simulink model "untitled"  (R2020b)
settings: Solver=FixedStepAuto  StartTime=0.0  StopTime=10.0  RelTol=1e-3
undefined symbols (not defined in the file): DiscIntNeverNeededParam
libraries: simulink x2
settings Model: Creator=xoxox  LastModifiedBy=xoxox
settings OptimizationCC: DefaultParameterBehavior=Inlined  EnhancedBackFolding=on  PassReuseOutputArgsAs=Individual arguments  ZeroExternalMemoryAtStartup=off  ZeroInternalMemoryAtStartup=off  OptimizeBlockOrder=speed  DifferentSizesBufferReuse=on  OptimizationCustomize=off  EfficientTunableParamExpr=on
settings DebuggingCC: ParameterTunabilityLossMsg=error
settings SFSimCC: MATLABDynamicMemAlloc=off
settings RTWCC: Description=Embedded Coder  SystemTargetFile=ert.tlc  GenCodeOnly=on  TemplateMakefile=ert_default_tmf  TargetLang=C++
settings CodeAppCC: ForceParamTrailComments=on  IgnoreCustomStorageClasses=off  OperatorAnnotations=on  SimulinkDataObjDesc=on  SFDataObjDesc=on  InsertBlockDesc=on
settings ERTTargetCC: TargetLangStandard=C++03 (ISO)  GenerateSampleERTMain=on  CodeInterfacePackaging=C++ class  InlinedParameterPlacement=NonHierarchical  RootIOFormat=Structure reference  ERTCustomFileTemplate=example_file_process.tlc

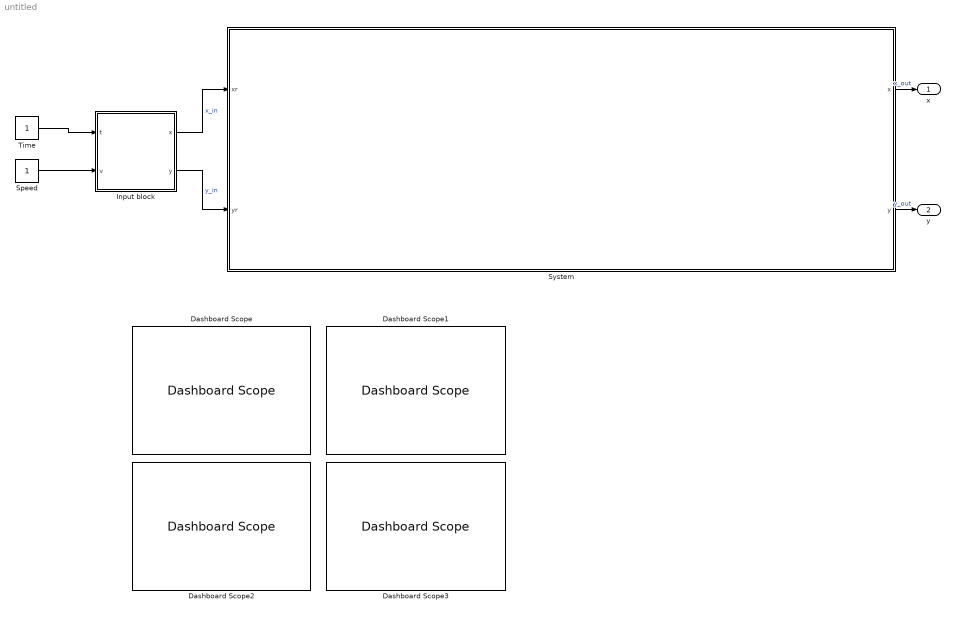
== system untitled ==
  Dashboard Scope{,1..3} (4 alike) : DashboardScope
  Input block : MATLAB Function  TreatAsAtomicUnit=on
  Speed : Constant
  System : Subsystem
  Time : Constant
  x : Outport  VectorParamsAs1DForOutWhenUnconnected=off
  y : Outport  Port=2  VectorParamsAs1DForOutWhenUnconnected=off
  wires:
  Input block/1(x) -> System/1(xr)  "x_in"
  Input block/2(y) -> System/2(yr)  "y_in"
  System/1(x) -> x/1  "x_out"
  System/2(y) -> y/1  "y_out"
  Speed/1 -> Input block/2(v)
  Time/1 -> Input block/1(t)

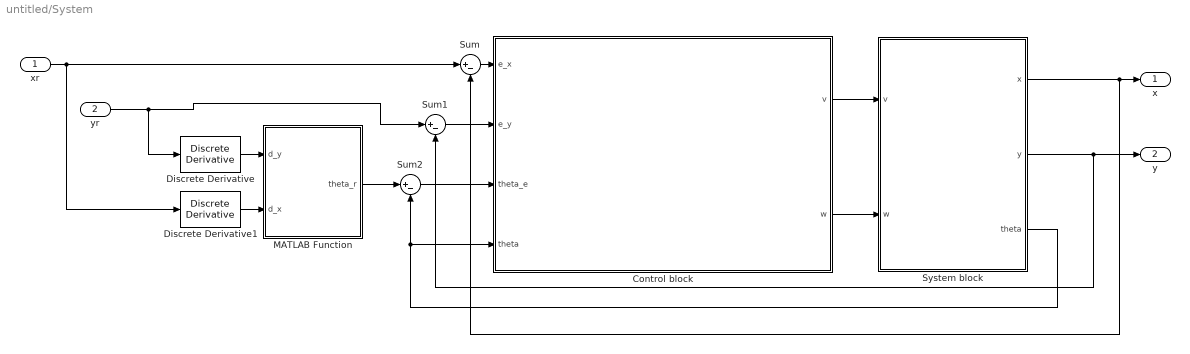
== system untitled/System ==
  xr : Inport
  yr : Inport  Port=2
  Control block : Subsystem
  Discrete Derivative : simulink/Discrete/Discrete Derivative  gainval=1.0  ICPrevScaledInput=0.0  OutMin=[]  OutMax=[]  OutDataType=fixdt(1, 16)  OutScaling=2^-10  DoSatur=off
  Discrete Derivative1 : simulink/Discrete/Discrete Derivative  gainval=1.0  ICPrevScaledInput=0.0  OutMin=[]  OutMax=[]  OutDataType=fixdt(1, 16)  OutScaling=2^-10  DoSatur=off
  MATLAB Function : MATLAB Function  TreatAsAtomicUnit=on
  Sum : Sum  Inputs=|+-
  Sum1 : Sum  Inputs=|+-
  Sum2 : Sum  Inputs=|+-
  System block : Subsystem
  x : Outport  VectorParamsAs1DForOutWhenUnconnected=off
  y : Outport  Port=2  VectorParamsAs1DForOutWhenUnconnected=off
  wires:
  Sum1/1 -> Control block/2(e_y)
  Control block/2(w) -> System block/2(w)
  Discrete Derivative/1 -> MATLAB Function/1(d_y)
  MATLAB Function/1(theta_r) -> Sum2/1
  System block/2(y) -> y/1, Sum1/2
  System block/3(theta) -> Control block/4(theta), Sum2/2
  System block/1(x) -> x/1, Sum/2
  Discrete Derivative1/1 -> MATLAB Function/2(d_x)
  Sum/1 -> Control block/1(e_x)
  Control block/1(v) -> System block/1(v)
  Sum2/1 -> Control block/3(theta_e)
  xr/1 -> Discrete Derivative1/1, Sum/1
  yr/1 -> Discrete Derivative/1, Sum1/1

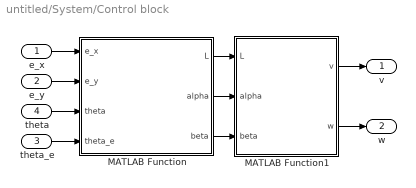
== system untitled/System/Control block ==
  e_x : Inport
  e_y : Inport  Port=2
  theta_e : Inport  Port=3
  theta : Inport  Port=4
  MATLAB Function : MATLAB Function  TreatAsAtomicUnit=on
  MATLAB Function1 : MATLAB Function  TreatAsAtomicUnit=on
  v : Outport  VectorParamsAs1DForOutWhenUnconnected=off
  w : Outport  Port=2  VectorParamsAs1DForOutWhenUnconnected=off
  wires:
  MATLAB Function1/1(v) -> v/1
  MATLAB Function1/2(w) -> w/1
  e_x/1 -> MATLAB Function/1(e_x)
  e_y/1 -> MATLAB Function/2(e_y)
  theta_e/1 -> MATLAB Function/4(theta_e)
  MATLAB Function/1(L) -> MATLAB Function1/1(L)
  MATLAB Function/2(alpha) -> MATLAB Function1/2(alpha)
  MATLAB Function/3(beta) -> MATLAB Function1/3(beta)
  theta/1 -> MATLAB Function/3(theta)

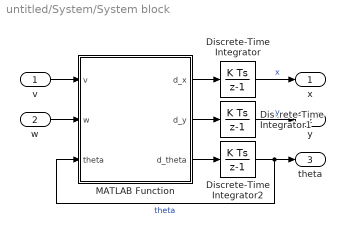
== system untitled/System/System block ==
  v : Inport
  w : Inport  Port=2
  Discrete-Time Integrator : DiscreteIntegrator  SampleTime=-1  ICPrevOutput=DiscIntNeverNeededParam  ICPrevScaledInput=DiscIntNeverNeededParam
  Discrete-Time Integrator1 : DiscreteIntegrator  SampleTime=-1  ICPrevOutput=DiscIntNeverNeededParam  ICPrevScaledInput=DiscIntNeverNeededParam
  Discrete-Time Integrator2 : DiscreteIntegrator  SampleTime=-1  ICPrevOutput=DiscIntNeverNeededParam  ICPrevScaledInput=DiscIntNeverNeededParam
  MATLAB Function : MATLAB Function  TreatAsAtomicUnit=on
  x : Outport  VectorParamsAs1DForOutWhenUnconnected=off
  y : Outport  Port=2  VectorParamsAs1DForOutWhenUnconnected=off
  theta : Outport  Port=3  VectorParamsAs1DForOutWhenUnconnected=off
  wires:
  Discrete-Time Integrator2/1 -> theta/1, MATLAB Function/3(theta)  "theta"
  MATLAB Function/1(d_x) -> Discrete-Time Integrator/1
  v/1 -> MATLAB Function/1(v)
  MATLAB Function/2(d_y) -> Discrete-Time Integrator1/1
  Discrete-Time Integrator/1 -> x/1  "x"
  w/1 -> MATLAB Function/2(w)
  Discrete-Time Integrator1/1 -> y/1  "y"
  MATLAB Function/3(d_theta) -> Discrete-Time Integrator2/1

== matlab function untitled/System/Control block/MATLAB Function ==
  data: e_x input; L output; e_y input; theta input; theta_e input; alpha output; beta output
function [L , alpha, beta] = to_parameters(e_x , e_y , theta , theta_e)
    L = sqrt(e_x * e_x + e_y * e_y);
    alpha = mod(atan2(e_y , e_x) , 2*pi) - theta;
    beta = theta_e - alpha;
end

== matlab function untitled/System/System block/MATLAB Function ==
  data: v input; d_x output; w input; theta input; d_y output; d_theta output
function [d_x,  d_y,  d_theta] = system(v , w , theta)

    d_x = v*cos(theta);
    d_y = v*sin(theta);
    d_theta = w;

end

== matlab function untitled/System/Control block/MATLAB Function1 ==
  data: L input; v output; w output; alpha input; beta input
function [v , w] = to_v_w(L, alpha , beta)

%old
% k_L = -3;
% k_alpha = -210;
% k_beta = 4.5;


k_L = -5.5;
k_alpha = -220;
k_beta = 2;

v = -k_L * L;
w = -k_alpha * alpha - k_beta * beta;

end

== matlab function untitled/System/MATLAB Function ==
  data: d_y input; d_x input; theta_r output
function theta_r = arctan2(d_y , d_x)
    theta_r = mod(atan2(d_y , d_x) , 2*pi);
end

== matlab function untitled/Input block ==
  data: x output; t input; y output; v input
function [x , y] = input(t , v)

    h = 10; %Straight line distance
    d = 5; %"Circle" diameter

    
    t = (mod(t , 2*h/v + 2*(d/v))); %% Loop

    is_on_part_1_flag = (t <= h/v);
    is_on_part_2_flag = (t > h/v && t <= h/v + d/v);
    is_on_part_3_flag = (t > h/v + d/v && t <= (2*h/v)+d/v); 
    is_on_part_4_flag = (~is_on_part_1_flag &&...
                         ~is_on_part_2_flag &&...
                         ~is_on_part_3_flag);
    
    timestamp = (is_on_part_1_flag) * t +...
                (is_on_part_2_flag) * (t - h/v) + ... 
                (is_on_part_3_flag) * (t - h/v - d/v)+...
                (is_on_part_4_flag) * (t - (2*h/v + (d/v)));


    y = is_on_part_1_flag * (timestamp*v)+...
        is_on_part_2_flag * (h + (d/2) * sin(pi*timestamp*v/d))+... 
        is_on_part_3_flag * (h-timestamp*v)+...
        is_on_part_4_flag * (-(d/2) * sin(pi*timestamp*v/d));

        
    x = is_on_part_1_flag * (0)+...
        is_on_part_2_flag * (timestamp*v)+... 
        is_on_part_3_flag * (d)+...
        is_on_part_4_flag * ((d - timestamp*v >0)*(d - timestamp*v));

            
            


end
